simulink model "Final_System"  (R2022b)
settings: Solver=FixedStepAuto  StartTime=0.0  StopTime=10.0  FixedStep=1e-3  RelTol=1e-3  EnableMultiTasking=on
undefined symbols (not defined in the file): ATR_Amp, ATR_CMP_DETECT, ATR_PULSE_WIDTH, ATR_RP, D0, D1, D10, D11, D12, D13, D2, D3, D4, D5, D6, D7, D8, D9, MODE, PERIOD, PTA0, PTA1, PTA2, PTB23, PTB9, PTC16, PTC17, PTC2, PTC3, PTC4, PTD0, PTD1, PTD2, PTD3, Sample_Amp, VENT_Amp, VENT_CMP_DETECT, VENT_PULSE_WIDTH, VENT_RP
libraries: frdmk64flib x27
settings Model: ExtModeTrigDuration=5  Creator=sarahalabdulrazzak  LastModifiedBy=sarahalabdulrazzak
settings SolverCC: AlgebraicLoopSolver=TrustRegion
settings OptimizationCC: EnhancedBackFolding=on  PassReuseOutputArgsAs=Individual arguments  ZeroExternalMemoryAtStartup=off  ZeroInternalMemoryAtStartup=off  MaxStackSize=64  OptimizeBlockOrder=speed  DifferentSizesBufferReuse=on  OptimizationCustomize=off  EfficientTunableParamExpr=on
settings DebuggingCC: ParameterTunabilityLossMsg=error  UnconnectedInputMsg=warning  UnconnectedOutputMsg=warning  UnconnectedLineMsg=warning  SFMachineParentedDataDiag=warning
settings HardwareCC: ProdBitPerPointer=32  ProdBitPerSizeT=32  ProdBitPerPtrDiffT=32  ProdLargestAtomicInteger=Long  ProdLargestAtomicFloat=Double  ProdWordSize=32  ProdHWDeviceType=ARM Compatible->ARM Cortex
settings ModelReferenceCC: EnableRefExpFcnMdlSchedulingChecks=on
settings SFSimCC: MATLABDynamicMemAlloc=off
settings RTWCC: Description=Embedded Coder  SystemTargetFile=ert.tlc  HardwareBoard=NXP FRDM-K64F  TLCOptions="-aInlineSetEventsForThisBaseRateFcn=TLC_FALSE -aSuppressMultiTaskScheduler=TLC_FALSE  -aRateBasedStepFcn=0"  TemplateMakefile=ert_default_tmf  Toolchain=GNU Tools for ARM Embedded Processors
settings CodeAppCC: ForceParamTrailComments=on  IgnoreCustomStorageClasses=off  OperatorAnnotations=on  SimulinkDataObjDesc=on  SFDataObjDesc=on  InsertBlockDesc=on

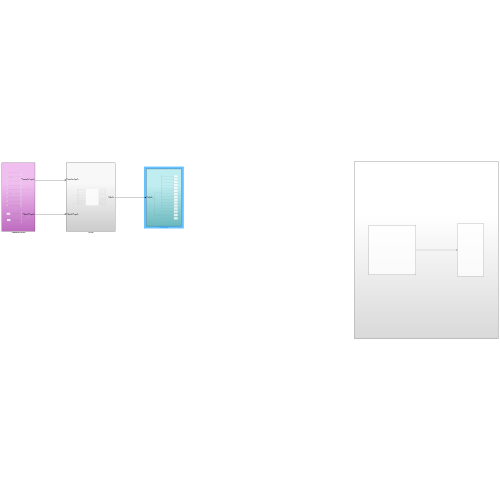
[thumbnail: Simulink's stored preview of the top-level diagram]
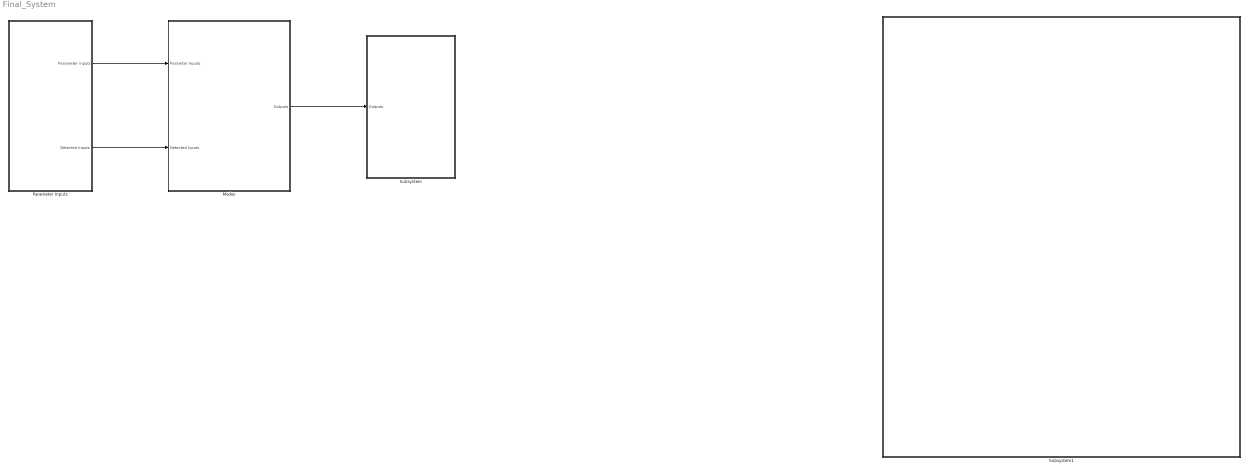
== system Final_System ==
  Modes : Subsystem
  Parameter Inputs : Subsystem
  Subsystem : Subsystem
  Subsystem1 : Subsystem
  wires:
  Parameter Inputs/1(Parameter Inputs) -> Modes/1(Paramter Inputs)
  Parameter Inputs/2(Detected Inputs) -> Modes/2(Detected Inputs)
  Modes/1("Outputs ") -> Subsystem/1("Outputs ")

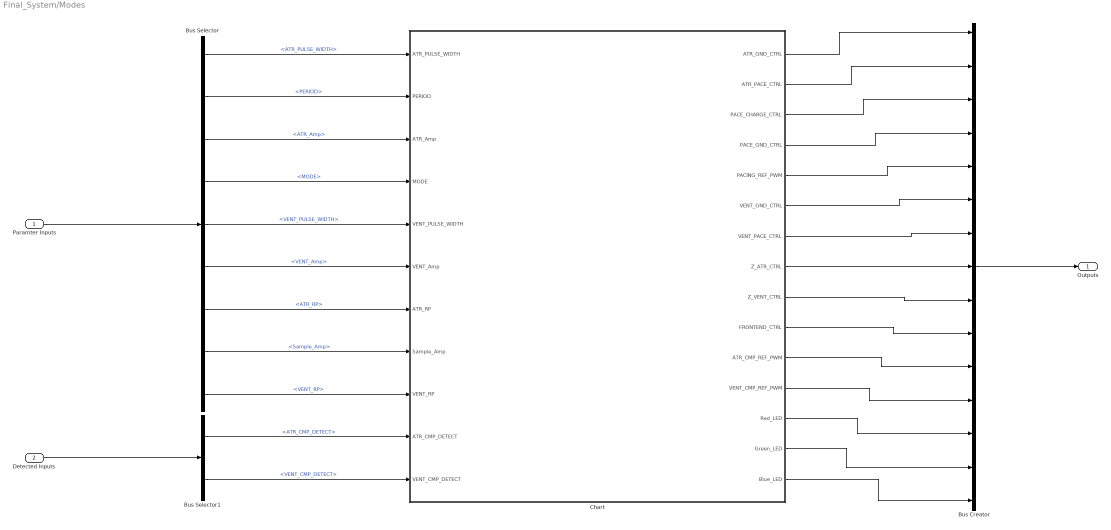
== system Final_System/Modes ==
  Paramter Inputs : Inport
  Detected Inputs : Inport  Port=2
  Bus Creator : BusCreator  Inputs=15
  Bus Selector : BusSelector  OutputSignals=ATR_PULSE_WIDTH,PERIOD,ATR_Amp,MODE,VENT_PULSE_WIDTH,VENT_Amp,ATR_RP,Sample_Amp,VENT_RP
  Bus Selector1 : BusSelector  OutputSignals=ATR_CMP_DETECT,VENT_CMP_DETECT
  Chart : Stateflow chart  TreatAsAtomicUnit=on
  "Outputs " : Outport
  wires:
  Paramter Inputs/1 -> Bus Selector/1
  Detected Inputs/1 -> Bus Selector1/1
  Bus Selector/4 -> Chart/4(MODE)  "<MODE>"
  Bus Selector/5 -> Chart/5(VENT_PULSE_WIDTH)  "<VENT_PULSE_WIDTH>"
  Bus Selector/6 -> Chart/6(VENT_Amp)  "<VENT_Amp>"
  Bus Selector/7 -> Chart/7(ATR_RP)  "<ATR_RP>"
  Bus Selector/8 -> Chart/8(Sample_Amp)  "<Sample_Amp>"
  Bus Selector/9 -> Chart/9(VENT_RP)  "<VENT_RP>"
  Bus Selector/1 -> Chart/1(ATR_PULSE_WIDTH)  "<ATR_PULSE_WIDTH>"
  Bus Selector/2 -> Chart/2(PERIOD)  "<PERIOD>"
  Bus Selector/3 -> Chart/3(ATR_Amp)  "<ATR_Amp>"
  Bus Selector1/1 -> Chart/10(ATR_CMP_DETECT)  "<ATR_CMP_DETECT>"
  Bus Selector1/2 -> Chart/11(VENT_CMP_DETECT)  "<VENT_CMP_DETECT>"
  Chart/1(ATR_GND_CTRL) -> Bus Creator/1
  Chart/2(ATR_PACE_CTRL) -> Bus Creator/2
  Chart/3(PACE_CHARGE_CTRL) -> Bus Creator/3
  Chart/4(PACE_GND_CTRL) -> Bus Creator/4
  Chart/5(PACING_REF_PWM) -> Bus Creator/5
  Chart/6(VENT_GND_CTRL) -> Bus Creator/6
  Chart/7(VENT_PACE_CTRL) -> Bus Creator/7
  Chart/8(Z_ATR_CTRL) -> Bus Creator/8
  Chart/9(Z_VENT_CTRL) -> Bus Creator/9
  Chart/10(FRONTEND_CTRL) -> Bus Creator/10
  Chart/11(ATR_CMP_REF_PWM) -> Bus Creator/11
  Chart/12(VENT_CMP_REF_PWM) -> Bus Creator/12
  Bus Creator/1 -> "Outputs "/1
  Chart/13(Red_LED) -> Bus Creator/13
  Chart/14(Green_LED) -> Bus Creator/14
  Chart/15(Blue_LED) -> Bus Creator/15

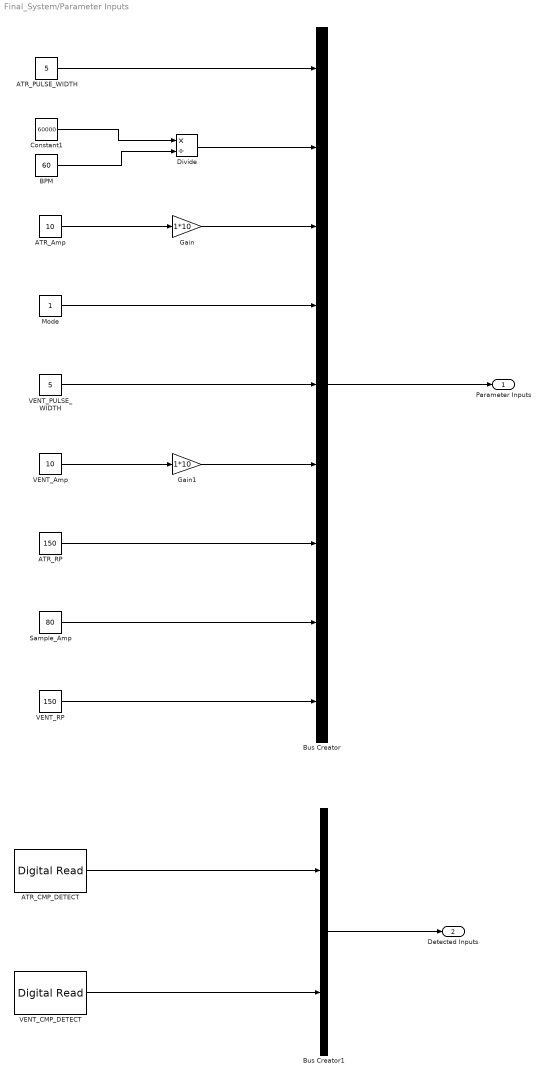
== system Final_System/Parameter Inputs ==
  ATR_Amp : Constant  Value=10
  ATR_CMP_DETECT : frdmk64flib/Digital Read  Whichpin=PTC16 (D0)  SampleTime=-1
  ATR_PULSE_WIDTH : Constant  Value=5
  ATR_RP : Constant  Value=150
  BPM : Constant  Value=60
  Bus Creator : BusCreator  Inputs=ATR_PULSE_WIDTH,PERIOD,ATR_Amp,MODE,VENT_PULSE_WIDTH,VENT_Amp,ATR_RP,Sample_Amp,VENT_RP
  Bus Creator1 : BusCreator  Inputs=ATR_CMP_DETECT,VENT_CMP_DETECT
  Constant1 : Constant  Value=60000
  Divide : Product  Inputs=*/
  Gain : Gain  Gain=1*10
  Gain1 : Gain  Gain=1*10
  Mode : Constant
  Sample_Amp : Constant  Value=80
  VENT_Amp : Constant  Value=10
  VENT_CMP_DETECT : frdmk64flib/Digital Read  Whichpin=PTC17 (D1)  SampleTime=-1
  VENT_PULSE_WIDTH : Constant  Value=5
  VENT_RP : Constant  Value=150
  Parameter Inputs : Outport
  Detected Inputs : Outport  Port=2
  wires:
  Bus Creator/1 -> Parameter Inputs/1
  ATR_PULSE_WIDTH/1 -> Bus Creator/1
  BPM/1 -> Divide/2
  Constant1/1 -> Divide/1
  Divide/1 -> Bus Creator/2
  ATR_Amp/1 -> Gain/1
  Gain/1 -> Bus Creator/3
  Mode/1 -> Bus Creator/4
  VENT_PULSE_WIDTH/1 -> Bus Creator/5
  VENT_Amp/1 -> Gain1/1
  Gain1/1 -> Bus Creator/6
  ATR_RP/1 -> Bus Creator/7
  Sample_Amp/1 -> Bus Creator/8
  VENT_RP/1 -> Bus Creator/9
  Bus Creator1/1 -> Detected Inputs/1
  VENT_CMP_DETECT/1 -> Bus Creator1/2
  ATR_CMP_DETECT/1 -> Bus Creator1/1

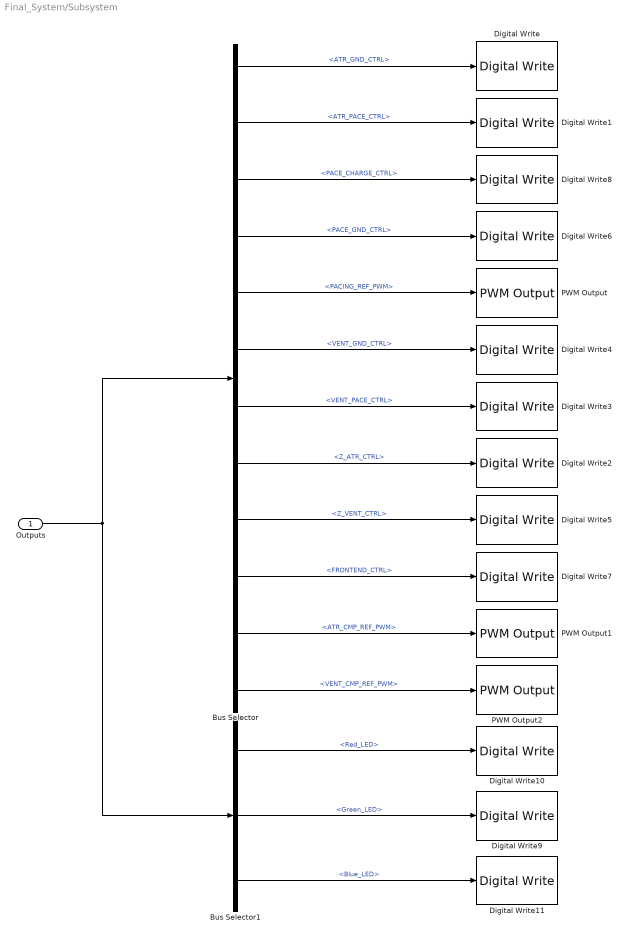
== system Final_System/Subsystem ==
  "Outputs " : Inport
  Bus Selector : BusSelector  OutputSignals=ATR_GND_CTRL,ATR_PACE_CTRL,PACE_CHARGE_CTRL,PACE_GND_CTRL,PACING_REF_PWM,VENT_GND_CTRL,VENT_PACE_CTRL,Z_ATR_CTRL,Z_VENT_CTRL,FRONTEND_CTRL,ATR_CMP_REF_PWM,VENT_CMP_REF_PWM
  Bus Selector1 : BusSelector  OutputSignals=Red_LED,Green_LED,Blue_LED
  Digital Write : frdmk64flib/Digital Write  Whichpin=PTD2 (D11)
  Digital Write1 : frdmk64flib/Digital Write  Whichpin=PTA0 (D8)
  Digital Write10 : frdmk64flib/Digital Write  Whichpin=RED_LED
  Digital Write11 : frdmk64flib/Digital Write  Whichpin=BLUE_LED
  Digital Write2 : frdmk64flib/Digital Write  Whichpin=PTB23 (D4)
  Digital Write3 : frdmk64flib/Digital Write  Whichpin=PTC4 (D9)
  Digital Write4 : frdmk64flib/Digital Write  Whichpin=PTD3 (D12)
  Digital Write5 : frdmk64flib/Digital Write  Whichpin=PTC3 (D7)
  Digital Write6 : frdmk64flib/Digital Write  Whichpin=PTD0 (D10)
  Digital Write7 : frdmk64flib/Digital Write  Whichpin=PTD1 (D13)
  Digital Write8 : frdmk64flib/Digital Write  Whichpin=PTB9 (D2)
  Digital Write9 : frdmk64flib/Digital Write  Whichpin=GREEN_LED
  PWM Output : frdmk64flib/PWM Output  Whichpin=PTA2 (D5)  InitialFrequency=2000  InitialDutyCycle=0
  PWM Output1 : frdmk64flib/PWM Output  Whichpin=PTC2 (D6)  InitialFrequency=2000  InitialDutyCycle=0
  PWM Output2 : frdmk64flib/PWM Output  Whichpin=PTA1 (D3)  InitialFrequency=2000  InitialDutyCycle=0
  wires:
  Bus Selector/1 -> Digital Write/1  "<ATR_GND_CTRL>"
  Bus Selector/2 -> Digital Write1/1  "<ATR_PACE_CTRL>"
  Bus Selector/3 -> Digital Write8/1  "<PACE_CHARGE_CTRL>"
  Bus Selector/4 -> Digital Write6/1  "<PACE_GND_CTRL>"
  Bus Selector/5 -> PWM Output/1  "<PACING_REF_PWM>"
  Bus Selector/6 -> Digital Write4/1  "<VENT_GND_CTRL>"
  Bus Selector/7 -> Digital Write3/1  "<VENT_PACE_CTRL>"
  Bus Selector/8 -> Digital Write2/1  "<Z_ATR_CTRL>"
  Bus Selector/9 -> Digital Write5/1  "<Z_VENT_CTRL>"
  Bus Selector/10 -> Digital Write7/1  "<FRONTEND_CTRL>"
  Bus Selector/11 -> PWM Output1/1  "<ATR_CMP_REF_PWM>"
  Bus Selector/12 -> PWM Output2/1  "<VENT_CMP_REF_PWM>"
  "Outputs "/1 -> Bus Selector/1, Bus Selector1/1
  Bus Selector1/1 -> Digital Write10/1  "<Red_LED>"
  Bus Selector1/2 -> Digital Write9/1  "<Green_LED>"
  Bus Selector1/3 -> Digital Write11/1  "<Blue_LED>"

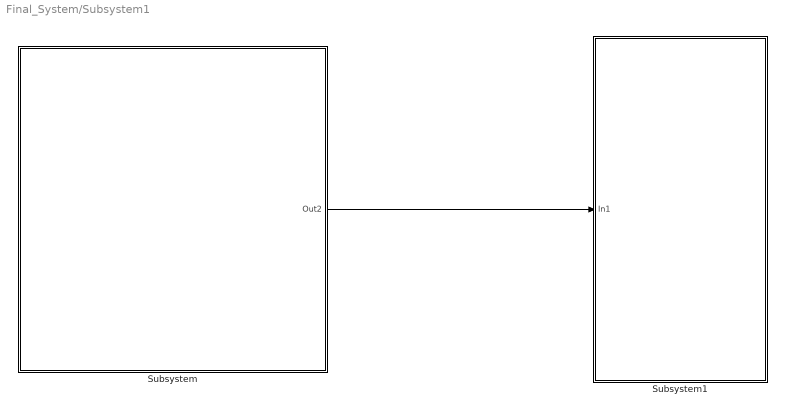
== system Final_System/Subsystem1 ==
  Subsystem : Subsystem
  Subsystem1 : Subsystem
  wires:
  Subsystem/1(Out2) -> Subsystem1/1(In1)

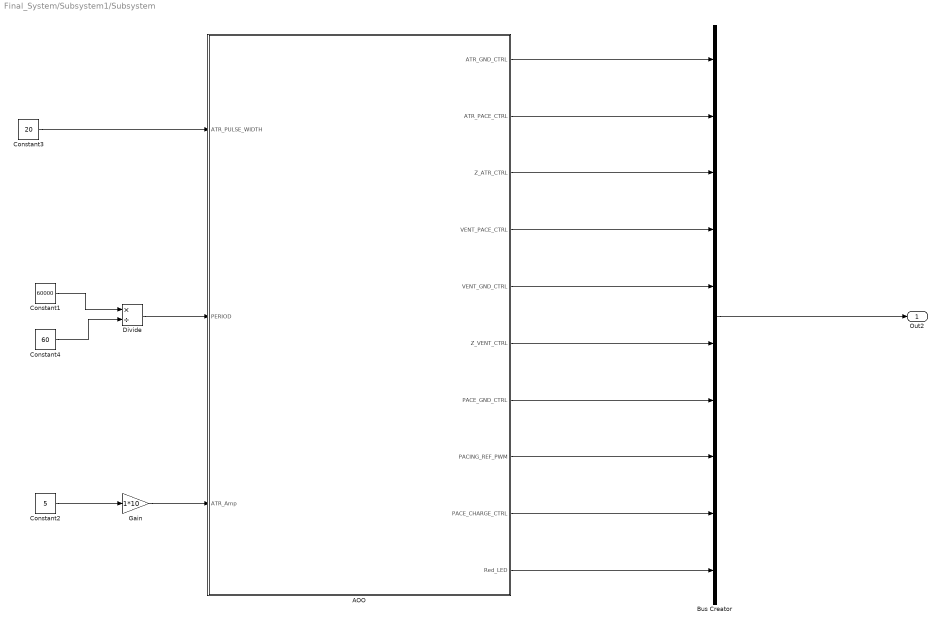
== system Final_System/Subsystem1/Subsystem ==
  AOO : Stateflow chart  TreatAsAtomicUnit=on
  Bus Creator : BusCreator  Inputs=10
  Constant1 : Constant  Value=60000
  Constant2 : Constant  Value=5
  Constant3 : Constant  Value=20
  Constant4 : Constant  Value=60
  Divide : Product  Inputs=*/
  Gain : Gain  Gain=1*10
  Out2 : Outport
  wires:
  Constant2/1 -> Gain/1
  Gain/1 -> AOO/3(ATR_Amp)
  Constant3/1 -> AOO/1(ATR_PULSE_WIDTH)
  AOO/4(VENT_PACE_CTRL) -> Bus Creator/4
  AOO/8(PACING_REF_PWM) -> Bus Creator/8
  Divide/1 -> AOO/2(PERIOD)
  AOO/3(Z_ATR_CTRL) -> Bus Creator/3
  AOO/5(VENT_GND_CTRL) -> Bus Creator/5
  Constant1/1 -> Divide/1
  AOO/9(PACE_CHARGE_CTRL) -> Bus Creator/9
  AOO/6(Z_VENT_CTRL) -> Bus Creator/6
  AOO/10(Red_LED) -> Bus Creator/10
  AOO/7(PACE_GND_CTRL) -> Bus Creator/7
  Constant4/1 -> Divide/2
  AOO/1(ATR_GND_CTRL) -> Bus Creator/1
  AOO/2(ATR_PACE_CTRL) -> Bus Creator/2
  Bus Creator/1 -> Out2/1

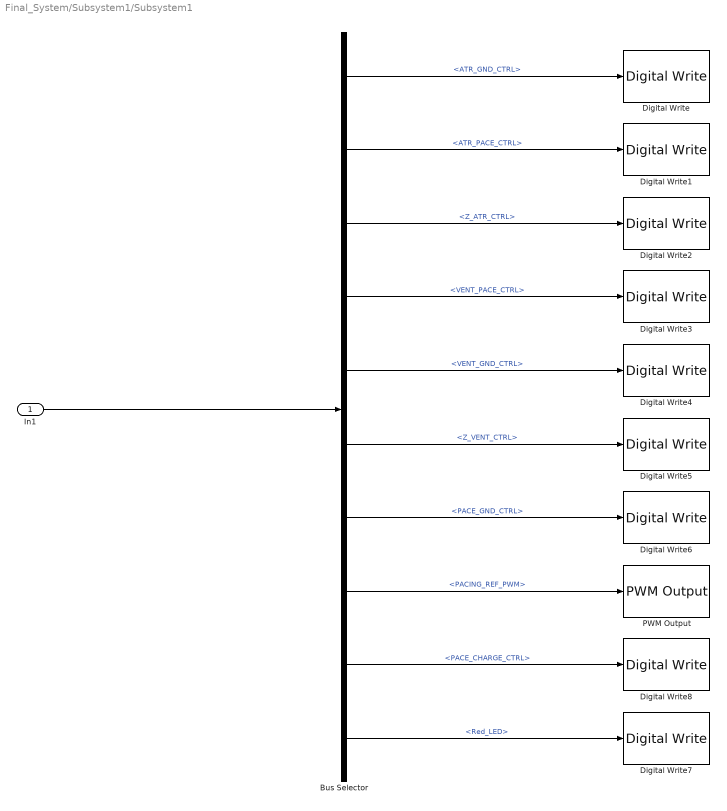
== system Final_System/Subsystem1/Subsystem1 ==
  In1 : Inport
  Bus Selector : BusSelector  OutputSignals=ATR_GND_CTRL,ATR_PACE_CTRL,Z_ATR_CTRL,VENT_PACE_CTRL,VENT_GND_CTRL,Z_VENT_CTRL,PACE_GND_CTRL,PACING_REF_PWM,PACE_CHARGE_CTRL,Red_LED
  Digital Write : frdmk64flib/Digital Write  Whichpin=PTD2 (D11)
  Digital Write1 : frdmk64flib/Digital Write  Whichpin=PTA0 (D8)
  Digital Write2 : frdmk64flib/Digital Write  Whichpin=PTB23 (D4)
  Digital Write3 : frdmk64flib/Digital Write  Whichpin=PTC4 (D9)
  Digital Write4 : frdmk64flib/Digital Write  Whichpin=PTD3 (D12)
  Digital Write5 : frdmk64flib/Digital Write  Whichpin=PTC3 (D7)
  Digital Write6 : frdmk64flib/Digital Write  Whichpin=PTD0 (D10)
  Digital Write7 : frdmk64flib/Digital Write  Whichpin=RED_LED
  Digital Write8 : frdmk64flib/Digital Write  Whichpin=PTB9 (D2)
  PWM Output : frdmk64flib/PWM Output  Whichpin=PTA2 (D5)  InitialFrequency=2000  InitialDutyCycle=0
  wires:
  In1/1 -> Bus Selector/1
  Bus Selector/1 -> Digital Write/1  "<ATR_GND_CTRL>"
  Bus Selector/2 -> Digital Write1/1  "<ATR_PACE_CTRL>"
  Bus Selector/3 -> Digital Write2/1  "<Z_ATR_CTRL>"
  Bus Selector/5 -> Digital Write4/1  "<VENT_GND_CTRL>"
  Bus Selector/4 -> Digital Write3/1  "<VENT_PACE_CTRL>"
  Bus Selector/6 -> Digital Write5/1  "<Z_VENT_CTRL>"
  Bus Selector/8 -> PWM Output/1  "<PACING_REF_PWM>"
  Bus Selector/9 -> Digital Write8/1  "<PACE_CHARGE_CTRL>"
  Bus Selector/10 -> Digital Write7/1  "<Red_LED>"
  Bus Selector/7 -> Digital Write6/1  "<PACE_GND_CTRL>"

== stateflow chart Final_System/Subsystem1/Subsystem/AOO ==
  state CHARGING
    entry:
    %Charge primary capcitor C22
    ATR_PACE_CTRL=LOW
    VENT_PACE_CTRL=LOW
    PACING_REF_PWM = ATR_Amp
    PACE_CHARGE_CTRL = HIGH
    %Discharge block capacitor C21
    PACE_GND_CTRL = HIGH
    %VENT_PACE_CTRL = LOW
    Z_ATR_CTRL = LOW
    Z_VENT_CTRL = LOW
    %ATR_PACE_CTRL = LOW
    ATR_GND_CTRL = HIGH
    VENT_GND_CTRL = LOW
    %use LED  to verify state
    Red_LED=false
  state DISCHARGING
    entry:
    %Discharge C22 primary capacitor
    %Charge C21 block capacitor
    PACE_CHARGE_CTRL = LOW
    PACE_GND_CTRL = HIGH
    ATR_PACE_CTRL = HIGH
    ATR_GND_CTRL = LOW
    Z_ATR_CTRL = LOW
    Z_VENT_CTRL = LOW
    VENT_GND_CTRL = LOW
    VENT_PACE_CTRL  = LOW
    PACING_REF_PWM = ATR_Amp
    %use LED  to verify state
    Red_LED=true
  (default) -> CHARGING
  CHARGING -> DISCHARGING : [after(PERIOD - ATR_PULSE_WIDTH,msec)]
  DISCHARGING -> CHARGING : [after(ATR_PULSE_WIDTH,msec)]
  data: ATR_GND_CTRL output; ATR_PACE_CTRL output; Z_ATR_CTRL output; VENT_PACE_CTRL output; VENT_GND_CTRL output; Z_VENT_CTRL output; PACE_GND_CTRL output; PACING_REF_PWM output; PACE_CHARGE_CTRL output; ATR_PULSE_WIDTH input; PERIOD input; HIGH local =true; LOW local =false; ATR_Amp input; Red_LED output

== stateflow chart Final_System/Modes/Chart ==
  state AOO
    entry:
    %Charge primary capcitor C22
    ATR_PACE_CTRL=LOW
    VENT_PACE_CTRL=LOW
    PACING_REF_PWM = ATR_Amp
    PACE_CHARGE_CTRL = HIGH
    %Discharge block capacitor C21
    PACE_GND_CTRL = HIGH
    %VENT_PACE_CTRL = LOW
    Z_ATR_CTRL = LOW
    Z_VENT_CTRL = LOW
    %ATR_PACE_CTRL = LOW
    ATR_GND_CTRL = HIGH
    VENT_GND_CTRL = LOW
    %use LED  to verify state
    Red_LED=false
    Green_LED=false
    Blue_LED=false
  state Identify_Mode_Path
    entry:
    % MODE = 1 (AOO)
    % MODE = 2 (AAI)
    % MODE = 3 (VOO)
    % MODE = 4 (VVI)
    %
    %pacemaker disconnected
    %stop sensing
    PACE_CHARGE_CTRL = LOW
    VENT_PACE_CTRL = LOW
    ATR_PACE_CTRL = LOW
    PACE_GND_CTRL = LOW
    ATR_GND_CTRL = LOW
    VENT_GND_CTRL = LOW
    Z_ATR_CTRL = LOW
    Z_VENT_CTRL = LOW
    FRONTEND_CTRL = LOW
  state AOO_ATR_PULSE
    entry:
    %Discharge C22 primary capacitor
    %Charge C21 block capacitor
    PACE_CHARGE_CTRL = LOW
    PACE_GND_CTRL = HIGH
    ATR_PACE_CTRL = HIGH
    ATR_GND_CTRL = LOW
    Z_ATR_CTRL = LOW
    Z_VENT_CTRL = LOW
    VENT_GND_CTRL = LOW
    VENT_PACE_CTRL  = LOW
    PACING_REF_PWM = ATR_Amp
    %use LED  to verify state
    Red_LED=true
    Green_LED=false
    Blue_LED=false
  state AAI
    entry:
    %sensing ON
    FRONTEND_CTRL = HIGH
    %Charge primary capcitor C22
    ATR_PACE_CTRL=LOW
    VENT_PACE_CTRL=LOW
    PACING_REF_PWM = ATR_Amp
    PACE_CHARGE_CTRL = HIGH
    %Discharge block capacitor C21
    PACE_GND_CTRL = HIGH
    VENT_PACE_CTRL = LOW
    Z_ATR_CTRL = LOW
    Z_VENT_CTRL = LOW
    ATR_GND_CTRL = HIGH
    VENT_GND_CTRL = LOW
    ATR_CMP_REF_PWM = Sample_Amp
    %use LED  to verify state
    Red_LED=false
    Blue_LED=false
    Green_LED=false
  state AAI_ATR_PULSE
    entry:
    %sensing OFF
    FRONTEND_CTRL = LOW
    %Discharge C22 primary capacitor
    %Charge C21 block capacitor
    PACE_CHARGE_CTRL = LOW
    PACE_GND_CTRL = HIGH
    ATR_PACE_CTRL = HIGH
    ATR_GND_CTRL = LOW
    Z_ATR_CTRL = LOW
    Z_VENT_CTRL = LOW
    VENT_GND_CTRL = LOW
    VENT_PACE_CTRL  = LOW
    PACING_REF_PWM = ATR_Amp
    %use LED  to verify state
    Red_LED=false
    Green_LED=false
    Blue_LED=true
  state VOO
    entry:
    %Charge primary capcitor C22
    ATR_PACE_CTRL=LOW
    VENT_PACE_CTRL=LOW
    PACING_REF_PWM = VENT_Amp
    PACE_CHARGE_CTRL = HIGH
    %Discharge block capacitor C21
    PACE_GND_CTRL = HIGH
    %VENT_PACE_CTRL = LOW
    Z_ATR_CTRL = LOW
    Z_VENT_CTRL = LOW
    %ATR_PACE_CTRL = LOW
    ATR_GND_CTRL = LOW
    VENT_GND_CTRL = HIGH
    %use LED  to verify state
    Red_LED=false
    Green_LED=false
    Blue_LED=false
  state VOO_VENT_PULSE
    entry:
    %Discharge C22 primary capacitor
    %Charge C21 block capacitor
    PACE_CHARGE_CTRL = LOW
    PACE_GND_CTRL = HIGH
    ATR_PACE_CTRL = LOW
    ATR_GND_CTRL = LOW
    Z_ATR_CTRL = LOW
    Z_VENT_CTRL = LOW
    VENT_GND_CTRL = LOW
    VENT_PACE_CTRL  = HIGH
    PACING_REF_PWM = VENT_Amp
    %use LED  to verify state
    Red_LED=false
    Green_LED=true
    Blue_LED=false
  state VVI
    entry:
    %sensing ON
    FRONTEND_CTRL = HIGH
    %Charge primary capcitor C22
    ATR_PACE_CTRL=LOW
    VENT_PACE_CTRL= LOW
    PACING_REF_PWM = VENT_Amp
    PACE_CHARGE_CTRL = HIGH
    %Discharge block capacitor C21
    PACE_GND_CTRL = HIGH
    VENT_PACE_CTRL = LOW
    Z_ATR_CTRL = LOW
    Z_VENT_CTRL = LOW
    ATR_GND_CTRL = LOW
    VENT_GND_CTRL = HIGH
    VENT_CMP_REF_PWM = Sample_Amp
    %use LED  to verify state
    Red_LED=true
    Green_LED=false
    Blue_LED=false
  state VVI_VENT_PULSE
    %sensing OFF
    FRONTEND_CTRL = LOW
    %Discharge C22 primary capacitor
    %Charge C21 block capacitor
    PACE_CHARGE_CTRL = LOW
    PACE_GND_CTRL = HIGH
    ATR_PACE_CTRL = LOW
    ATR_GND_CTRL = LOW
    Z_ATR_CTRL = LOW
    Z_VENT_CTRL = LOW
    VENT_GND_CTRL = LOW
    VENT_PACE_CTRL  = HIGH
    PACING_REF_PWM = VENT_Amp
    %use LED  to verify state
    Red_LED=false
    Green_LED=true
    Blue_LED=false
  (default) -> Identify_Mode_Path
  AOO -> AOO_ATR_PULSE : [after(PERIOD - ATR_PULSE_WIDTH,msec)]
  Identify_Mode_Path -> AOO [order 1] : [MODE == 1]
  AOO_ATR_PULSE -> AOO : [after(ATR_PULSE_WIDTH,msec)]
  AAI_ATR_PULSE -> AAI : after(ATR_PULSE_WIDTH,msec)
  Identify_Mode_Path -> AAI [order 2] : [MODE == 2]
  AAI -> (junction 41)
  (junction 41) -> AAI_ATR_PULSE [order 1] : after(PERIOD - ATR_PULSE_WIDTH,msec)[ATR_CMP_DETECT == LOW]
  (junction 41) -> (junction 35) [order 2] : [ATR_CMP_DETECT == HIGH]
  (junction 35) -> AAI : after(ATR_RP, msec)
  VOO -> VOO_VENT_PULSE : after(PERIOD - VENT_PULSE_WIDTH,msec)
  Identify_Mode_Path -> VOO [order 3] : [MODE == 3]
  VOO_VENT_PULSE -> VOO : after(VENT_PULSE_WIDTH,msec)
  VVI_VENT_PULSE -> VVI : after(VENT_PULSE_WIDTH,msec)
  Identify_Mode_Path -> VVI [order 4] : [MODE == 4]
  VVI -> (junction 61)
  (junction 61) -> VVI_VENT_PULSE [order 1] : after(PERIOD - VENT_PULSE_WIDTH,msec)[VENT_CMP_DETECT == LOW]
  (junction 61) -> (junction 59) [order 2] : [VENT_CMP_DETECT == HIGH]
  (junction 59) -> VVI : after(VENT_RP, msec)
  data: ATR_PULSE_WIDTH input; PERIOD input; ATR_Amp input; MODE input; VENT_PULSE_WIDTH input; VENT_Amp input; ATR_RP input; Sample_Amp input; VENT_RP input; ATR_CMP_DETECT input; VENT_CMP_DETECT input; HIGH local =1; LOW local =0; ATR_GND_CTRL output; ATR_PACE_CTRL output; PACE_CHARGE_CTRL output; PACE_GND_CTRL output; PACING_REF_PWM output; VENT_GND_CTRL output; VENT_PACE_CTRL output; Z_ATR_CTRL output; Z_VENT_CTRL output; FRONTEND_CTRL output; ATR_CMP_REF_PWM output; VENT_CMP_REF_PWM output; Red_LED output; Green_LED output; Blue_LED output
